simulink model "example1_pid"  (R2023b)
settings: Solver=FixedStepAuto  StartTime=0.0  StopTime=20  FixedStep=Ts  RelTol=1e-3
values from neighbouring files (symbols this model uses):
  J = 0.02    [example1_pid.m]
  Kb = 0.1    [example1_pid.m]
  Kf = 0.01    [example1_pid.m]
  KI = 1    [example1_pid.m]
  Km = 1    [example1_pid.m]
  L = 0.5    [example1_pid.m]
  R = 2    [example1_pid.m]
settings Model: ExtModeTrigDuration=2  Creator=FM23  LastModifiedBy=FM23
settings OptimizationCC: EnhancedBackFolding=on  PassReuseOutputArgsAs=Individual arguments  ZeroExternalMemoryAtStartup=off  ZeroInternalMemoryAtStartup=off  MaxStackSize=64  OptimizeBlockOrder=speed  DifferentSizesBufferReuse=on  OptimizationCustomize=off  EfficientTunableParamExpr=on
settings DebuggingCC: ParameterTunabilityLossMsg=error
settings HardwareCC: ProdBitPerInt=16  ProdBitPerPointer=16  ProdBitPerSizeT=16  ProdBitPerPtrDiffT=16  ProdLargestAtomicFloat=None  ProdWordSize=8  ProdHWDeviceType=Atmel->AVR
settings SFSimCC: MATLABDynamicMemAlloc=off
settings RTWCC: Description=Embedded Coder  SystemTargetFile=ert.tlc  HardwareBoard=Arduino Mega 2560  TemplateMakefile=ert_default_tmf  Toolchain=Arduino AVR  BuildConfiguration=Faster Runs
settings CodeAppCC: ForceParamTrailComments=on  IgnoreCustomStorageClasses=off  OperatorAnnotations=on  SimulinkDataObjDesc=on  SFDataObjDesc=on  InsertBlockDesc=on
settings ERTTargetCC: SupportContinuousTime=on  SupportVariableSizeSignals=on  ExtModeTransport=3  ExtModeStaticAlloc=on  ExtModeAutomaticAllocSize=off  ExtModeStaticAllocSize=2048  ExtModeMexFile=ext_xcp  ExtModeIntrfLevel=Level2 - Open

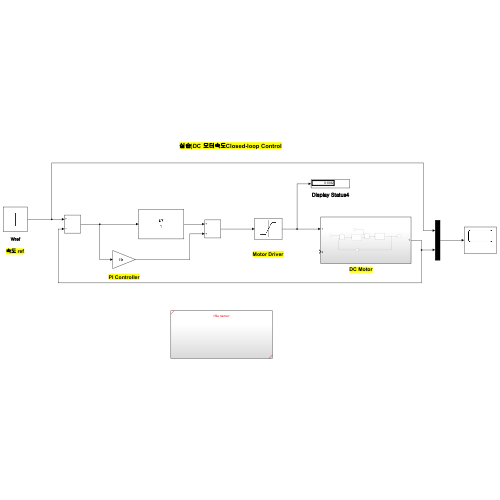
[thumbnail: Simulink's stored preview of the top-level diagram]
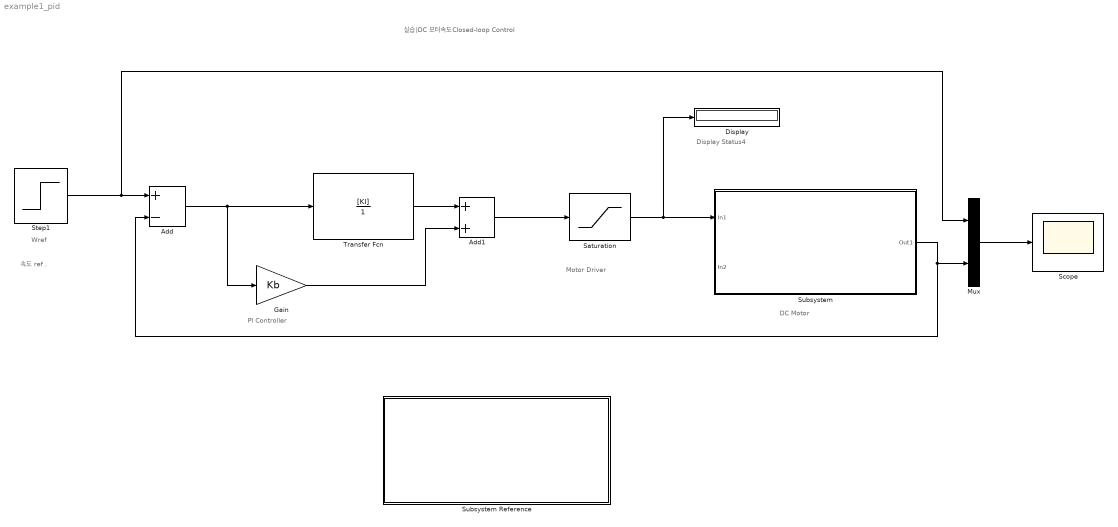
== system example1_pid ==
  note: 실습)DC 모터속도Closed-loop Control
  note: 속도 ref .
  note: Display Status4
  note: Wref
  note: DC Motor
  note: PI Controller
  note: Motor Driver
  Add : Sum  Inputs=+-
  Add1 : Sum
  Display : Display
  Gain : Gain  Gain=Kb
  Mux : Mux  Inputs=2
  Saturation : Saturate
  Scope : Scope
  Step1 : Step  After=100  SampleTime=0
  Subsystem : Subsystem
  Subsystem Reference : Subsystem  ReferencedSubsystem=<file name>
  Transfer Fcn : TransferFcn  Numerator=[KI]  Denominator=[1]
  wires:
  Step1/1 -> Mux/1, Add/1
  Add/1 -> Gain/1, Transfer Fcn/1
  Transfer Fcn/1 -> Add1/1
  Gain/1 -> Add1/2
  Mux/1 -> Scope/1
  Subsystem/1(Out1) -> Add/2, Mux/2
  Add1/1 -> Saturation/1
  Saturation/1 -> Display/1, Subsystem/1(In1)

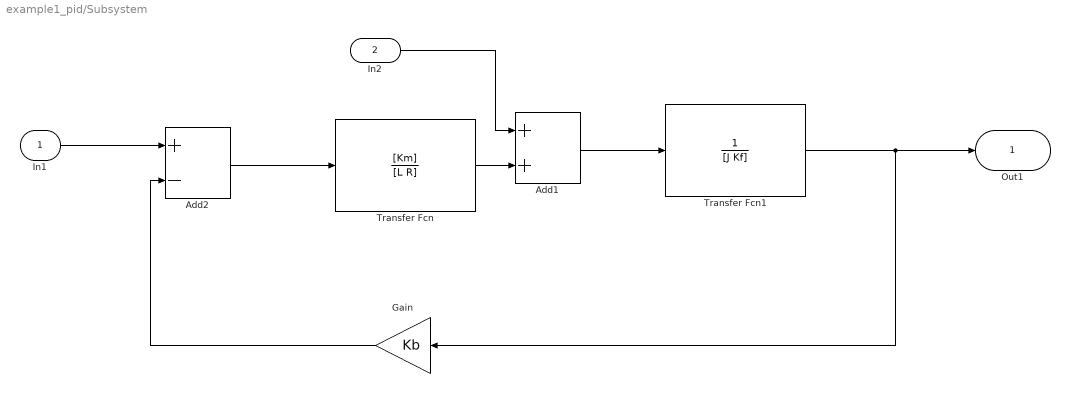
== system example1_pid/Subsystem ==
  In1 : Inport
  In2 : Inport  Port=2
  Add1 : Sum
  Add2 : Sum  Inputs=+-
  Gain : Gain  Gain=Kb
  Transfer Fcn : TransferFcn  Numerator=[Km]  Denominator=[L R]
  Transfer Fcn1 : TransferFcn  Denominator=[J Kf]
  Out1 : Outport
  wires:
  Transfer Fcn1/1 -> Out1/1, Gain/1
  In1/1 -> Add2/1
  Add2/1 -> Transfer Fcn/1
  Transfer Fcn/1 -> Add1/2
  In2/1 -> Add1/1
  Gain/1 -> Add2/2
  Add1/1 -> Transfer Fcn1/1

== system example1_pid/Subsystem Reference ==
